simulink model "sampleModel1481"  (R2023a)
settings: Solver=VariableStepAuto  StartTime=0.0  StopTime=10.0  RelTol=1e-3
libraries: hdlsllib x6, simulink x1
settings Model: Creator=user1  LastModifiedBy=user1

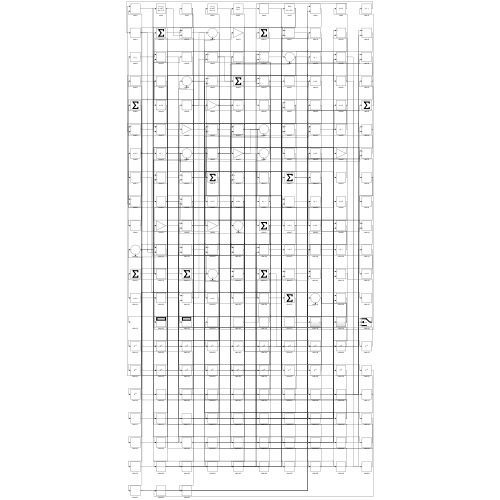
[thumbnail: Simulink's stored preview of the top-level diagram]
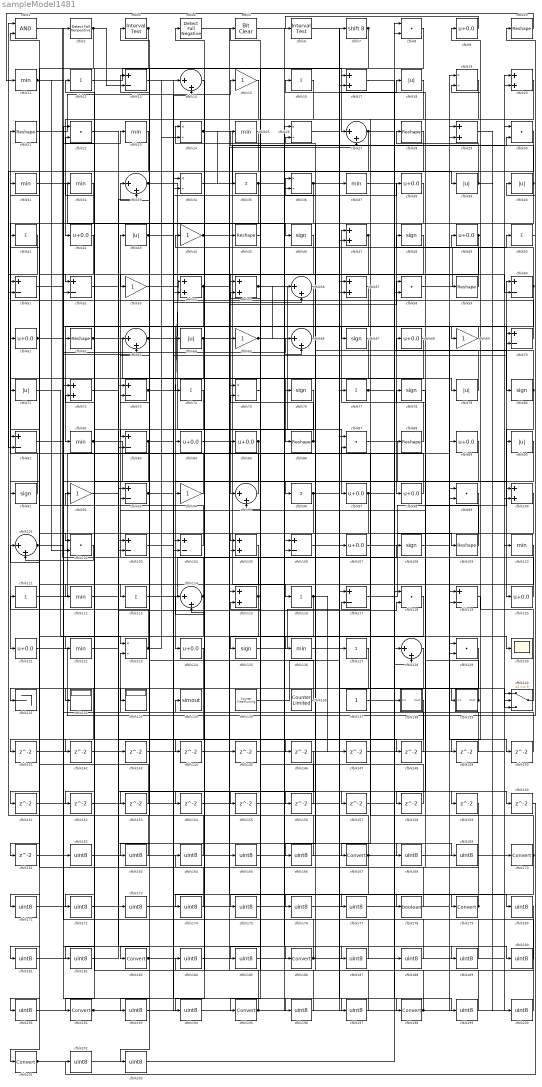
== system sampleModel1481 ==
  cfblk1 : Logic  AllPortsSameDT=off  OutDataTypeStr=boolean
  cfblk{10,21,28,45,59,62,86,88,109} (9 alike) : Reshape
  cfblk{17,20,29,47,54..55,57,72,100,105,115} (11 alike) : Sum
  cfblk{14,27,33,56,63,66,95,101,114,128} (10 alike) : Sum  Inputs=|++
  cfblk{8,22,30,58,87,99,102,118,129} (9 alike) : DotProduct  OutDataTypeStr=Inherit: Inherit via internal rule
  cfblk{13,51..52,60,70,73,81,83,93,103..104,106,117,119} (14 alike) : Sum  Inputs=+-
  cfblk{9,38,42,49,61,68,84..85,89,97..98,107,120..121,124} (15 alike) : Bias  Bias=0.0  SaturateOnIntegerOverflow=off
  cfblk{46,48,67,76,78,80,91,108,125} (9 alike) : Signum
  cfblk{11,23,25,31..32,37,82,110,112,122,126} (11 alike) : MinMax
  cfblk{12,16,35,41,50,74,77,96,111,113,116,127} (12 alike) : Sum  Inputs=+
  cfblk{19,24,26,34,36,75,123} (7 alike) : Product  Inputs=*/  RndMeth=Zero  SaturateOnIntegerOverflow=on
  cfblk130 : Scope
  cfblk131 : Terminator
  cfblk132 : Display
  cfblk133 : Display
  cfblk134 : ToWorkspace  VariableName=simout  SaveFormat=Timeseries  SampleTime=-1
  cfblk135 : hdlsllib/Sources/Counter Free-Running  NumBits=16  tsamp=-1
  cfblk136 : hdlsllib/Sources/Counter Limited  uplimit=7  tsamp=-1
  cfblk137 : Constant  SampleTime=-1
  cfblk138 : Subsystem
      settings: LibrarySourceBlock=|
      | hdlsllib/Ports &
      | Subsystems/Subsystem
  cfblk139 : Subsystem
      settings: LibrarySourceBlock=|
      | hdlsllib/Ports &
      | Subsystems/Subsystem
  cfblk140 : Switch  SaturateOnIntegerOverflow=off  InputSameDT=off
  cfblk{141..161} (21 alike) : Delay  SampleTime=1
  cfblk{15,44,53,65,69,92,94} (7 alike) : Gain
  cfblk{162..166,168..169,171..177,180..182,184..185,187..191,193..194,196..197,199..200,202..203} (32 alike) : DataTypeConversion  OutDataTypeStr=uint8  SaturateOnIntegerOverflow=off  RndMeth=Floor
  cfblk{167,170,179,183,186,192,195,198,201} (9 alike) : DataTypeConversion  SaturateOnIntegerOverflow=off  RndMeth=Floor
  cfblk178 : DataTypeConversion  OutDataTypeStr=boolean  SaturateOnIntegerOverflow=off  RndMeth=Floor
  cfblk{18,39..40,43,64,71,79,90} (8 alike) : Abs  SaturateOnIntegerOverflow=off
  cfblk2 : hdlsllib/Logic and Bit Operations/Detect Fall Nonpositive  vinit=0  OutDataTypeStr=boolean
  cfblk3 : hdlsllib/Logic and Bit Operations/Interval Test  IntervalClosedRight=on  uplimit=0.5  IntervalClosedLeft=on  lowlimit=-0.5  OutDataTypeStr=boolean
  cfblk4 : hdlsllib/Logic and Bit Operations/Detect Fall Negative  vinit=0  OutDataTypeStr=boolean
  cfblk5 : simulink/Logic and Bit Operations/Bit Clear  iBit=0
      settings: LibrarySourceBlock=|
      | hdlsllib/Logic and Bit
      | Operations/Bit Clear
  cfblk6 : hdlsllib/Logic and Bit Operations/Interval Test  IntervalClosedRight=on  uplimit=0.5  IntervalClosedLeft=on  lowlimit=-0.5  OutDataTypeStr=boolean
  cfblk7 : ArithShift  BitShiftNumber=8
  wires:
  cfblk15/1 -> cfblk42/1
  cfblk88/1 -> cfblk47/1
  cfblk114/1 -> cfblk2/1, cfblk73/2, cfblk133/1
  cfblk22/1 -> cfblk186/1
  cfblk53/1 -> cfblk79/1
  cfblk12/1 -> cfblk27/1
  cfblk24/1 -> cfblk116/1, cfblk35/1
  cfblk75/1 -> cfblk195/1
  cfblk47/1 -> cfblk95/1, cfblk83/2
  cfblk48/1 -> cfblk52/1
  cfblk67/1 -> cfblk124/1
  cfblk71/1 -> cfblk123/1
  cfblk36/1 -> cfblk121/1, cfblk159/1
  cfblk68/1 -> cfblk86/1
  cfblk85/1 -> cfblk94/1, cfblk154/1
  cfblk89/1 -> cfblk123/2
  cfblk107/1 -> cfblk109/1
  cfblk120/1 -> cfblk43/1
  cfblk55/1 -> cfblk97/1, cfblk119/2
  cfblk56/1 -> cfblk84/1
  cfblk27/1 -> cfblk138/1(In1), cfblk51/2, cfblk102/1
  cfblk37/1 -> cfblk98/1
  cfblk94/1 -> cfblk12/1
  cfblk117/1 -> cfblk60/1
  cfblk91/1 -> cfblk21/1
  cfblk33/1 -> cfblk117/1, cfblk60/2
  cfblk2/1 -> cfblk52/2, cfblk13/2
  cfblk121/1 -> cfblk40/1
  cfblk54/1 -> cfblk82/1, cfblk178/1
  cfblk95/1 -> cfblk61/1
  cfblk31/1 -> cfblk46/1
  cfblk79/1 -> cfblk36/1
  cfblk113/1 -> cfblk108/1
  cfblk40/1 -> cfblk25/1, cfblk114/2
  cfblk5/1 -> cfblk179/1
  cfblk28/1 -> cfblk125/1
  cfblk116/1 -> cfblk147/1, cfblk194/1
  cfblk42/1 -> cfblk71/1
  cfblk59/1 -> cfblk48/1
  cfblk20/1 -> cfblk167/1
  cfblk125/1 -> cfblk107/1
  cfblk58/1 -> cfblk50/1
  cfblk38/1 -> cfblk126/1
  cfblk35/1 -> cfblk113/1, cfblk39/1
  cfblk111/1 -> cfblk19/1
  cfblk101/1 -> cfblk63/2, cfblk196/1
  cfblk65/1 -> cfblk56/1, cfblk148/1
  cfblk32/1 -> cfblk81/1
  cfblk62/1 -> cfblk76/1, cfblk87/1
  cfblk73/1 -> cfblk54/1, cfblk70/2
  cfblk139/1(Out1) -> cfblk93/2, cfblk16/1
  cfblk80/1 -> cfblk120/1, cfblk24/1, cfblk90/1
  cfblk19/1 -> cfblk36/2
  cfblk21/1 -> cfblk15/1
  cfblk128/1 -> cfblk201/1
  cfblk39/1 -> cfblk28/1, cfblk200/1
  cfblk11/1 -> cfblk96/1, cfblk102/2
  cfblk49/1 -> cfblk53/1, cfblk19/2
  cfblk41/1 -> cfblk81/2
  cfblk83/1 -> cfblk132/1, cfblk38/1
  cfblk3/1 -> cfblk62/1, cfblk91/1
  cfblk72/1 -> cfblk33/2
  cfblk63/1 -> cfblk127/1, cfblk56/2
  cfblk136/1 -> cfblk3/1
  cfblk93/1 -> cfblk64/1, cfblk14/2
  cfblk18/1 -> cfblk54/2
  cfblk81/1 -> cfblk66/1
  cfblk29/1 -> cfblk170/1
  cfblk109/1 -> cfblk68/1
  cfblk60/1 -> cfblk44/1, cfblk156/1
  cfblk16/1 -> cfblk112/1
  cfblk66/1 -> cfblk65/1
  cfblk84/1 -> cfblk119/1
  cfblk26/1 -> cfblk198/1
  cfblk70/1 -> cfblk51/1
  cfblk61/1 -> cfblk69/1, cfblk187/1
  cfblk50/1 -> cfblk10/1
  cfblk6/1 -> cfblk139/1(In1)
  cfblk96/1 -> cfblk18/1, cfblk161/1, cfblk193/1
  cfblk74/1 -> cfblk122/1
  cfblk44/1 -> cfblk80/1, cfblk45/1
  cfblk115/1 -> cfblk72/2, cfblk181/1
  cfblk43/1 -> cfblk14/1, cfblk197/1
  cfblk123/1 -> cfblk111/1, cfblk24/2
  cfblk137/1 -> cfblk49/1
  cfblk57/1 -> cfblk192/1
  cfblk102/1 -> cfblk101/2
  cfblk14/1 -> cfblk74/1
  cfblk51/1 -> cfblk23/1
  cfblk10/1 -> cfblk11/1
  cfblk135/1 -> cfblk77/1
  cfblk87/1 -> cfblk100/1
  cfblk64/1 -> cfblk130/1, cfblk58/1, cfblk27/2, cfblk191/1
  cfblk82/1 -> cfblk115/1, cfblk157/1
  cfblk98/1 -> cfblk13/1
  cfblk77/1 -> cfblk140/3, cfblk199/1
  cfblk45/1 -> cfblk105/1
  cfblk97/1 -> cfblk105/2, cfblk70/1
  cfblk112/1 -> cfblk118/2
  cfblk76/1 -> cfblk104/2
  cfblk7/1 -> cfblk17/1, cfblk83/1
  cfblk99/1 -> cfblk183/1
  cfblk34/1 -> cfblk30/2
  cfblk140/1 -> cfblk9/1
  cfblk86/1 -> cfblk55/2, cfblk166/1
  cfblk69/1 -> cfblk67/1
  cfblk104/1 -> cfblk31/1
  cfblk105/1 -> cfblk131/1
  cfblk9/1 -> cfblk6/1
  cfblk118/1 -> cfblk141/1
  cfblk141/1 -> cfblk34/2
  cfblk129/1 -> cfblk142/1
  cfblk52/1 -> cfblk143/1
  cfblk143/1 -> cfblk30/1
  cfblk110/1 -> cfblk144/1
  cfblk144/1 -> cfblk114/1
  cfblk145/1 -> cfblk140/2
  cfblk122/1 -> cfblk146/1
  cfblk147/1 -> cfblk117/2
  cfblk148/1 -> cfblk73/1
  cfblk119/1 -> cfblk149/1
  cfblk149/1 -> cfblk72/1
  cfblk108/1 -> cfblk150/1
  cfblk150/1 -> cfblk33/1
  cfblk138/1(Out1) -> cfblk151/1
  cfblk151/1 -> cfblk47/2
  cfblk23/1 -> cfblk152/1
  cfblk152/1 -> cfblk93/1
  cfblk127/1 -> cfblk153/1
  cfblk153/1 -> cfblk101/1
  cfblk154/1 -> cfblk17/2
  cfblk90/1 -> cfblk155/1
  cfblk156/1 -> cfblk115/2
  cfblk78/1 -> cfblk158/1
  cfblk158/1 -> cfblk95/2
  cfblk126/1 -> cfblk160/1
  cfblk161/1 -> cfblk58/2
  cfblk1/1 -> cfblk162/1
  cfblk162/1 -> cfblk7/1
  cfblk146/1 -> cfblk163/1
  cfblk163/1 -> cfblk1/1
  cfblk159/1 -> cfblk164/1
  cfblk164/1 -> cfblk1/2
  cfblk4/1 -> cfblk165/1
  cfblk165/1 -> cfblk85/1
  cfblk166/1 -> cfblk4/1
  cfblk167/1 -> cfblk63/1, cfblk140/1, cfblk177/1
  cfblk142/1 -> cfblk168/1
  cfblk168/1 -> cfblk20/1
  cfblk17/1 -> cfblk169/1
  cfblk169/1 -> cfblk20/2
  cfblk170/1 -> cfblk87/2, cfblk185/1
  cfblk46/1 -> cfblk171/1
  cfblk171/1 -> cfblk29/1
  cfblk124/1 -> cfblk172/1
  cfblk172/1 -> cfblk29/2
  cfblk92/1 -> cfblk173/1
  cfblk173/1 -> cfblk129/2
  cfblk25/1 -> cfblk174/1
  cfblk174/1 -> cfblk92/1
  cfblk8/1 -> cfblk175/1
  cfblk175/1 -> cfblk129/1
  cfblk13/1 -> cfblk176/1
  cfblk176/1 -> cfblk8/1
  cfblk177/1 -> cfblk8/2
  cfblk178/1 -> cfblk5/1
  cfblk179/1 -> cfblk41/1, cfblk78/1
  cfblk103/1 -> cfblk180/1
  cfblk181/1 -> cfblk103/1
  cfblk100/1 -> cfblk182/1
  cfblk182/1 -> cfblk103/2
  cfblk183/1 -> cfblk145/1, cfblk110/1
  cfblk180/1 -> cfblk184/1
  cfblk184/1 -> cfblk99/1
  cfblk185/1 -> cfblk99/2
  cfblk186/1 -> cfblk55/1, cfblk89/1
  cfblk187/1 -> cfblk22/1
  cfblk157/1 -> cfblk188/1
  cfblk188/1 -> cfblk22/2
  cfblk106/1 -> cfblk189/1
  cfblk189/1 -> cfblk34/1
  cfblk155/1 -> cfblk190/1
  cfblk190/1 -> cfblk106/1
  cfblk191/1 -> cfblk106/2
  cfblk192/1 -> cfblk66/2, cfblk104/1
  cfblk193/1 -> cfblk57/1
  cfblk194/1 -> cfblk57/2
  cfblk195/1 -> cfblk37/1, cfblk59/1, cfblk134/1
  cfblk196/1 -> cfblk75/1
  cfblk197/1 -> cfblk75/2
  cfblk198/1 -> cfblk100/2, cfblk32/1
  cfblk199/1 -> cfblk26/1
  cfblk200/1 -> cfblk26/2
  cfblk201/1 -> cfblk88/1, cfblk118/1
  cfblk160/1 -> cfblk202/1
  cfblk202/1 -> cfblk128/1
  cfblk30/1 -> cfblk203/1
  cfblk203/1 -> cfblk128/2

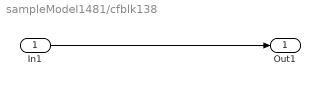
== system sampleModel1481/cfblk138 ==
  In1 : Inport
  Out1 : Outport
  wires:
  In1/1 -> Out1/1

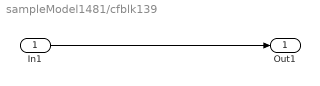
== system sampleModel1481/cfblk139 ==
  In1 : Inport
  Out1 : Outport
  wires:
  In1/1 -> Out1/1
